simulink model "gtm_design"  (Simulink 9.1)
settings: Solver=ode3  StartTime=0.0  StopTime=Inf  FixedStep=Timestep  MaxStep=.1  RelTol=1e-5
InitFcn:
  | if ~exist('MAG3TempComp','var')
  |     appendmws(Cal_params_T2)
  | end
StopFcn:
  | MWSout=grabmws(bdroot);
  | MWSout.lastrun=datestr(now);
model workspace: external: MATLAB Code tmpfile_simWS.mat (data not in the file)
undefined symbols (not defined in the file or in its folder): bias, Timestep, WindDir, WindSpd
libraries: aeroutilslib x2, simulink x2, aircraft_lib x1
CloseFcn:
  | rtwprivate ssgensfun ModelCloseRequest gtm_design
settings Model: Creator=cox  LastModifiedBy=E183308  ExtModeAutoUpdateStatusClock=off
settings DataIOCC: LimitDataPoints=on  MaxDataPoints=50000  SaveFormat=Structure  SignalLoggingSaveFormat=ModelDataLogs  SaveOutput=off  SignalLogging=off
settings OptimizationCC: BooleanDataType=off  ExpressionDepthLimit=2147483647  InitFltsAndDblsToZero=on
settings DebuggingCC: SaveWithParameterizedLinksMsg=none  SignalResolutionControl=TryResolveAllWithWarning  InheritedTsInSrcMsg=none  MultiTaskDSMMsg=warning  MultiTaskCondExecSysMsg=none  FcnCallInpInsideContextMsg=warning  StateNameClashWarn=warning
settings HardwareCC: TargetHWDeviceType=32-bit Generic
settings GRTTargetCC: TargetFcnLib=ansi_tfl_tmw.mat

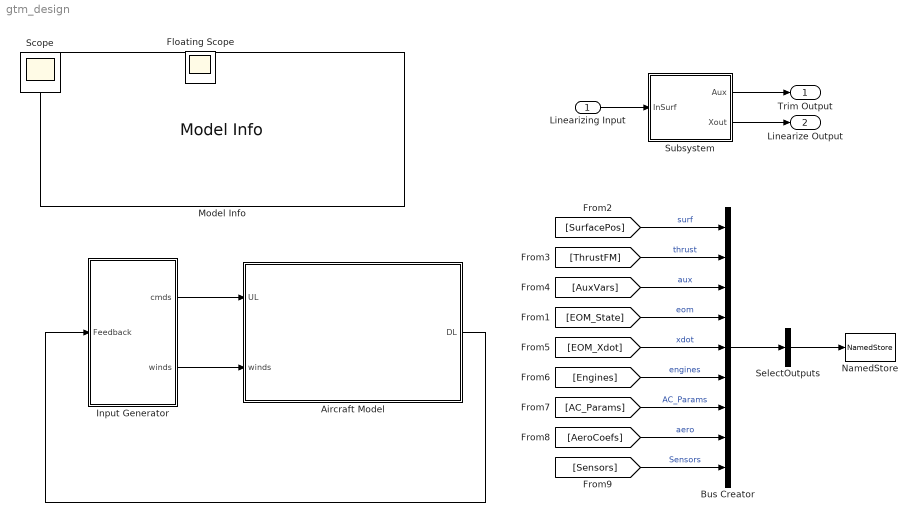
== system gtm_design ==
  Linearizing Input : Inport
  Aircraft Model : Subsystem  BlockChoice=GTM_T2
      link override GTM_T2/Avionics: BlockChoice=Blank
      link override GTM_T2/Engines/GTM_T2/Bypass: Value=0
      link override GTM_T2/Sensors: BlockChoice=GTM_T2 gtm_design
      link override L1011_S2/Avionics: BlockChoice=Blank
      link override L1011_S2/Sensors: BlockChoice=Blank
      settings: AttributesFormatString=%<BlockChoice>  TemplateBlock=aircraft_lib/Aircraft Model  MemberBlocks=GTM_T2,L1011_S2
  Bus Creator : BusCreator  Inputs=9
  Input Generator : Subsystem  AncestorBlock=UserContent_lib/Input Generator
  Model Info : simulink/Model-Wide Utilities/Model Info  Frame=on  DisplayStringWithTags=|  HorizontalTextAlignment=Center  LeftAlignmentValue=0.5
      | GTM Design-Simulation Model
      | Subversion Info: %<ModelVersion>
      | Last modified by %<LastModifiedBy> on %<LastModificationDate>
      | 
      | Copyright 2009
      | United States Government as represented by the 
      | Administrator of the National and Aeronautics and Space Administration.
      | 
      | No copyright is claimed in the United States under Title 17, U.S. Code.
      | All Other Rights Reserved.
  NamedStore : aeroutilslib/NamedStore  Npts=inf  VarName=sout  expand=off
  SelectOutputs : BusSelector  OutputSignals=aux.eas,aux.alpha,aux.beta,aux.gamma  OutputAsBus=on
  Subsystem : Subsystem
  Trim Output : Outport
  Linearize Output : Outport  Port=2
  Floating Scope : Scope
  Scope : Scope
  wires:
  SelectOutputs/1 -> NamedStore/1
  [SurfacePos] -> Bus Creator/1  "surf"
  Linearizing Input/1 -> Subsystem/1(InSurf)
  Subsystem/1(Aux) -> Trim Output/1
  [EOM_State] -> Bus Creator/4  "eom"
  [AuxVars] -> Bus Creator/3  "aux"
  [ThrustFM] -> Bus Creator/2  "thrust"
  Subsystem/2(Xout) -> Linearize Output/1
  [EOM_Xdot] -> Bus Creator/5  "xdot"
  [Engines] -> Bus Creator/6  "engines"
  [AC_Params] -> Bus Creator/7  "AC_Params"
  Bus Creator/1 -> SelectOutputs/1
  Input Generator/1(cmds) -> Aircraft Model/1(UL)
  Input Generator/2(winds) -> Aircraft Model/2(winds)
  Aircraft Model/1(DL) -> Input Generator/1(Feedback)
  [AeroCoefs] -> Bus Creator/8  "aero"
  [Sensors] -> Bus Creator/9  "Sensors"

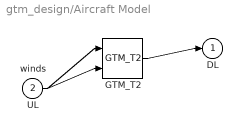
== system gtm_design/Aircraft Model ==
  UL : Inport
  winds : Inport  Port=2
  GTM_T2 : aircraft_lib/GTM_T2  Tag=From trunk/GTMsim/gtm_model.mdl revision 162  SystemSampleTime=-1
  DL : Outport
  wires:
  UL/1 -> GTM_T2/1
  winds/1 -> GTM_T2/2
  GTM_T2/1 -> DL/1

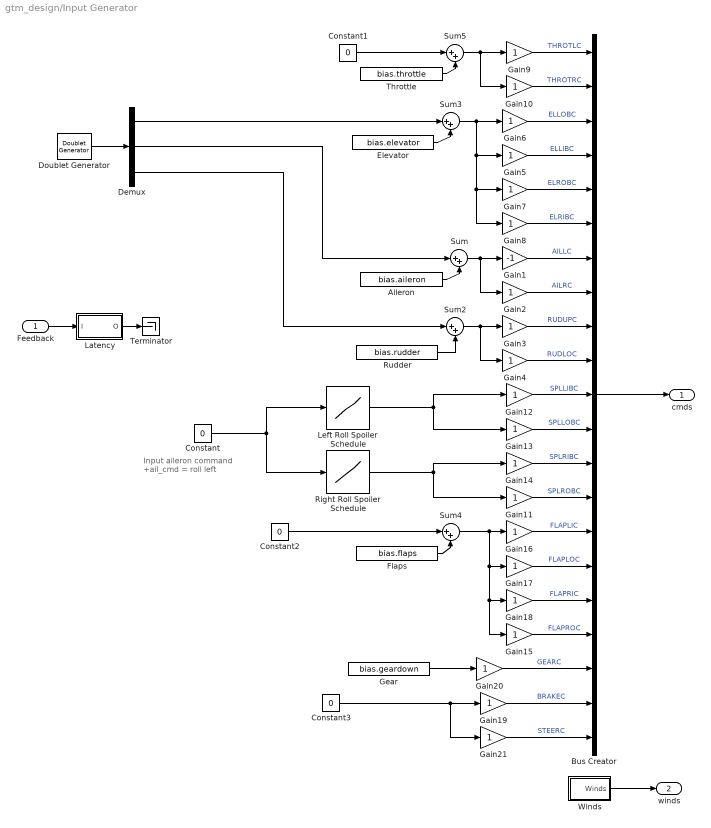
== system gtm_design/Input Generator ==
  note: Input aileron command
      | +ail_cmd = roll left
  Feedback : Inport
  Aileron : Constant  Value=bias.aileron
  Bus Creator : BusCreator  Inputs=21
  Constant{,1..3} (4 alike) : Constant  Value=0
  Demux : Demux  Outputs=3
  Doublet Generator : aeroutilslib/Doublet Generator  timeon=[2 12 7]  pulsewidth=[0.5 0.5 0.5]  amplitude=[0 0 0]
  Elevator : Constant  Value=bias.elevator
  Flaps : Constant  Value=bias.flaps
  Gain1 : Gain  Gain=-1  SaturateOnIntegerOverflow=on  OutDataTypeStr=Inherit: Same as input  ParamDataTypeStr=Inherit: Same as input
  Gain{2..21} (20 alike) : Gain  SaturateOnIntegerOverflow=on  OutDataTypeStr=Inherit: Same as input  ParamDataTypeStr=Inherit: Same as input
  Gear : Constant  Value=bias.geardown
  Latency : Subsystem
  Left Roll Spoiler Schedule : Lookup  InputValues="[-20\t-11.76\t-2.36\t0\t2.36\t11.76\t20\t]"  Table=[0 0 0 0 0 9 45]  LookUpMeth=Interpolation-Use End Values
  Right Roll Spoiler Schedule : Lookup  InputValues="[-20\t-11.76\t-2.36\t0\t2.36\t11.76\t20\t]"  Table=[45 9 0 0 0 0 0]  LookUpMeth=Interpolation-Use End Values
  Rudder : Constant  Value=bias.rudder
  Sum{,2..5} (5 alike) : Sum  Inputs=|++
  Terminator : Terminator
  Throttle : Constant  Value=bias.throttle
  Winds : Subsystem
  cmds : Outport
  winds : Outport  Port=2
  wires:
  Latency/1(O) -> Terminator/1
  Winds/1(Winds) -> winds/1
  Constant/1 -> Right Roll Spoiler Schedule/1, Left Roll Spoiler Schedule/1
  Right Roll Spoiler Schedule/1 -> Gain11/1, Gain14/1
  Left Roll Spoiler Schedule/1 -> Gain13/1, Gain12/1
  Gain12/1 -> Bus Creator/11  "SPLLIBC"
  Gain13/1 -> Bus Creator/12  "SPLLOBC"
  Gain14/1 -> Bus Creator/13  "SPLRIBC"
  Gain11/1 -> Bus Creator/14  "SPLROBC"
  Gain16/1 -> Bus Creator/15  "FLAPLIC"
  Gain17/1 -> Bus Creator/16  "FLAPLOC"
  Gain18/1 -> Bus Creator/17  "FLAPRIC"
  Gain15/1 -> Bus Creator/18  "FLAPROC"
  Gain9/1 -> Bus Creator/1  "THROTLC"
  Gain10/1 -> Bus Creator/2  "THROTRC"
  Gain5/1 -> Bus Creator/4  "ELLIBC"
  Gain6/1 -> Bus Creator/3  "ELLOBC"
  Gain7/1 -> Bus Creator/5  "ELROBC"
  Gain8/1 -> Bus Creator/6  "ELRIBC"
  Gain1/1 -> Bus Creator/7  "AILLC"
  Gain2/1 -> Bus Creator/8  "AILRC"
  Gain3/1 -> Bus Creator/9  "RUDUPC"
  Gain4/1 -> Bus Creator/10  "RUDLOC"
  Throttle/1 -> Sum5/2
  Constant1/1 -> Sum5/1
  Sum5/1 -> Gain10/1, Gain9/1
  Sum3/1 -> Gain6/1, Gain5/1, Gain7/1, Gain8/1
  Aileron/1 -> Sum/2
  Elevator/1 -> Sum3/2
  Sum/1 -> Gain1/1, Gain2/1
  Sum2/1 -> Gain3/1, Gain4/1
  Rudder/1 -> Sum2/2
  Flaps/1 -> Sum4/2
  Constant2/1 -> Sum4/1
  Sum4/1 -> Gain16/1, Gain17/1, Gain18/1, Gain15/1
  Doublet Generator/1 -> Demux/1
  Demux/2 -> Sum/1
  Demux/3 -> Sum2/1
  Gain19/1 -> Bus Creator/20  "BRAKEC"
  Gear/1 -> Gain20/1
  Constant3/1 -> Gain19/1, Gain21/1
  Demux/1 -> Sum3/1
  Bus Creator/1 -> cmds/1
  Feedback/1 -> Latency/1(I)
  Gain20/1 -> Bus Creator/19  "GEARC"
  Gain21/1 -> Bus Creator/21  "STEERC"

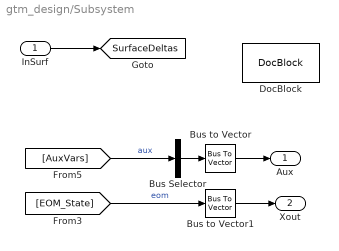
== system gtm_design/Subsystem ==
  InSurf : Inport
  Bus Selector : BusSelector  OutputSignals=eas,tas,alpha,beta,gamma,gndtrack  OutputAsBus=on
  Bus to Vector : BusToVector
  Bus to Vector1 : BusToVector
  DocBlock : simulink/Model-Wide Utilities/DocBlock  DocumentType=Text
      content=|
      | Inputs and Outputs selected here have a specific ordering.
      |
      |
      |
      | Do not change this without also changing output channel ordering in associated linmodel.m and
      | trimgtm.m functions
  Aux : Outport
  Xout : Outport  Port=2
  tag scope: SurfaceDeltas=global
  wires:
  [AuxVars] -> Bus Selector/1  "aux"
  [EOM_State] -> Bus to Vector1/1  "eom"
  Bus Selector/1 -> Bus to Vector/1
  InSurf/1 -> [SurfaceDeltas]
  Bus to Vector/1 -> Aux/1
  Bus to Vector1/1 -> Xout/1

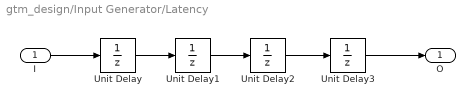
== system gtm_design/Input Generator/Latency ==
  I : Inport
  Unit Delay{,1..3} (4 alike) : UnitDelay  SampleTime=Timestep
  O : Outport
  wires:
  Unit Delay3/1 -> O/1
  Unit Delay2/1 -> Unit Delay3/1
  Unit Delay1/1 -> Unit Delay2/1
  Unit Delay/1 -> Unit Delay1/1
  I/1 -> Unit Delay/1

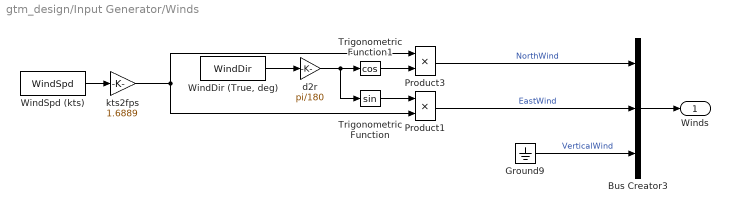
== system gtm_design/Input Generator/Winds ==
  Bus Creator3 : BusCreator  Inputs=3
  Ground9 : Ground
  Product1 : Product  Inputs=**  SaturateOnIntegerOverflow=on  InputSameDT=on  OutDataTypeStr=Inherit: Same as first input
  Product3 : Product  Inputs=**  SaturateOnIntegerOverflow=on  InputSameDT=on  OutDataTypeStr=Inherit: Same as first input
  Trigonometric Function : Trigonometry
  Trigonometric Function1 : Trigonometry  Operator=cos
  "WindDir (True, deg)" : Constant  Value=WindDir
  WindSpd (kts) : Constant  Value=WindSpd
  d2r : Gain  Gain=pi/180  SaturateOnIntegerOverflow=on  OutDataTypeStr=Inherit: Same as input  ParamDataTypeStr=Inherit: Same as input
  kts2fps : Gain  Gain=1.6889  SaturateOnIntegerOverflow=on  OutDataTypeStr=Inherit: Same as input  ParamDataTypeStr=Inherit: Same as input
  Winds : Outport
  wires:
  kts2fps/1 -> Product1/2, Product3/1
  WindSpd (kts)/1 -> kts2fps/1
  "WindDir (True, deg)"/1 -> d2r/1
  d2r/1 -> Trigonometric Function1/1, Trigonometric Function/1
  Trigonometric Function1/1 -> Product3/2
  Trigonometric Function/1 -> Product1/1
  Bus Creator3/1 -> Winds/1
  Ground9/1 -> Bus Creator3/3  "VerticalWind"
  Product1/1 -> Bus Creator3/2  "EastWind"
  Product3/1 -> Bus Creator3/1  "NorthWind"
